simulink model "npc_controller"  (R2022a)
settings: Solver=FixedStepDiscrete  StartTime=0.0  StopTime=20  RelTol=1e-3  EnableMultiTasking=on
undefined symbols (not defined in the file): CAN_O_INT, CANA_BASE, Down, GPTRIP1SEL, GPTRIP2SEL, GPTRIP3SEL, Tsw, TZ1, TZ2, TZ3, Up
libraries: simulink x147, hdlsllib x90, c2802xlib x34, c2837xDlib x20, c280xlib x12, canmsglib x9, c2838xlib x8, idelinklib_common x3, c2806xlib x2, slpidlib x2, c28004xlib x2, c281xlib x2
(part 12 of 42)

== system npc_controller/CONTROL/STATE-MACHINE/CPU_CONTROL_200_A2_precharge_pfc_ok2/updateSequencePhA/pol_ix1 ==
  note: 75dig -> 3iac
  ix : Inport
  Trigger : TriggerPort  TriggerType=function-call  VariantControl=(inherit)  PortDimensions=1
  If : If  IfExpression="(u1 > -8)  & (u1 < 8)"  ElseIfExpressions=u1 >= 8
  Merge : Merge  Inputs=3
  neg : Subsystem  TreatAsAtomicUnit=on
  pos : Subsystem  TreatAsAtomicUnit=on
  zero : Subsystem  TreatAsAtomicUnit=on
  pol_ix : Outport
  wires:
  ix/1 -> If/1
  If/1 -> zero/Action
  zero/1(Out1) -> Merge/1
  If/2 -> pos/Action
  If/3 -> neg/Action
  neg/1(Out1) -> Merge/3
  pos/1(Out1) -> Merge/2
  Merge/1 -> pol_ix/1

== system npc_controller/CONTROL/STATE-MACHINE/CPU_CONTROL_200_A2_precharge_pfc_ok2/updateSequencePhA/pol_vxn1 ==
  note: 16dig -> 5vac
  vxn : Inport
  Trigger : TriggerPort  TriggerType=function-call  VariantControl=(inherit)  PortDimensions=1
  If : If  IfExpression="(u1 > -16)  & (u1 < 16)"  ElseIfExpressions=u1 >= 16
  Merge : Merge  Inputs=3
  neg : Subsystem  TreatAsAtomicUnit=on
  pos : Subsystem  TreatAsAtomicUnit=on
  zero : Subsystem  TreatAsAtomicUnit=on
  pol_vxn : Outport
  wires:
  Merge/1 -> pol_vxn/1
  pos/1(Out1) -> Merge/2
  neg/1(Out1) -> Merge/3
  If/3 -> neg/Action
  If/2 -> pos/Action
  zero/1(Out1) -> Merge/1
  If/1 -> zero/Action
  vxn/1 -> If/1

== system npc_controller/CONTROL/STATE-MACHINE/CPU_CONTROL_200_A2_precharge_pfc_ok2/updateSequencePhB/pol_final1 ==
  vxn : Inport
  ix : Inport  Port=2
  Trigger : TriggerPort  TriggerType=function-call  VariantControl=(inherit)  PortDimensions=1
  If : If  NumInputs=2  IfExpression="((u1 == 1)  & (u2 == 2)) | ((u1 == 2)  & (u2 == 1))"
  Merge : Merge
  pol_vxn : Subsystem  TreatAsAtomicUnit=on
  prot : Subsystem  TreatAsAtomicUnit=on
  pol : Outport
  wires:
  ix/1 -> If/2
  vxn/1 -> pol_vxn/1(vxn), If/1
  Merge/1 -> pol/1
  If/2 -> pol_vxn/Action
  prot/1(Out1) -> Merge/1
  If/1 -> prot/Action
  pol_vxn/1(Out1) -> Merge/2

== system npc_controller/CONTROL/STATE-MACHINE/CPU_CONTROL_200_A2_precharge_pfc_ok2/updateSequencePhB/pol_ix1 ==
  note: 75dig -> 3iac
  ix : Inport
  Trigger : TriggerPort  TriggerType=function-call  VariantControl=(inherit)  PortDimensions=1
  If : If  IfExpression="(u1 > -8)  & (u1 < 8)"  ElseIfExpressions=u1 >= 8
  Merge : Merge  Inputs=3
  neg : Subsystem  TreatAsAtomicUnit=on
  pos : Subsystem  TreatAsAtomicUnit=on
  zero : Subsystem  TreatAsAtomicUnit=on
  pol_ix : Outport
  wires:
  ix/1 -> If/1
  If/1 -> zero/Action
  zero/1(Out1) -> Merge/1
  If/2 -> pos/Action
  If/3 -> neg/Action
  neg/1(Out1) -> Merge/3
  pos/1(Out1) -> Merge/2
  Merge/1 -> pol_ix/1

== system npc_controller/CONTROL/STATE-MACHINE/CPU_CONTROL_200_A2_precharge_pfc_ok2/updateSequencePhB/pol_vxn1 ==
  note: 16dig -> 5vac
  vxn : Inport
  Trigger : TriggerPort  TriggerType=function-call  VariantControl=(inherit)  PortDimensions=1
  If : If  IfExpression="(u1 > -16)  & (u1 < 16)"  ElseIfExpressions=u1 >= 16
  Merge : Merge  Inputs=3
  neg : Subsystem  TreatAsAtomicUnit=on
  pos : Subsystem  TreatAsAtomicUnit=on
  zero : Subsystem  TreatAsAtomicUnit=on
  pol_vxn : Outport
  wires:
  Merge/1 -> pol_vxn/1
  pos/1(Out1) -> Merge/2
  neg/1(Out1) -> Merge/3
  If/3 -> neg/Action
  If/2 -> pos/Action
  zero/1(Out1) -> Merge/1
  If/1 -> zero/Action
  vxn/1 -> If/1

== system npc_controller/CONTROL/STATE-MACHINE/CPU_CONTROL_200_A2_precharge_pfc_ok2/updateSequencePhC/pol_final1 ==
  vxn : Inport
  ix : Inport  Port=2
  Trigger : TriggerPort  TriggerType=function-call  VariantControl=(inherit)  PortDimensions=1
  If : If  NumInputs=2  IfExpression="((u1 == 1)  & (u2 == 2)) | ((u1 == 2)  & (u2 == 1))"
  Merge : Merge
  pol_vxn : Subsystem  TreatAsAtomicUnit=on
  prot : Subsystem  TreatAsAtomicUnit=on
  pol : Outport
  wires:
  ix/1 -> If/2
  vxn/1 -> pol_vxn/1(vxn), If/1
  Merge/1 -> pol/1
  If/2 -> pol_vxn/Action
  prot/1(Out1) -> Merge/1
  If/1 -> prot/Action
  pol_vxn/1(Out1) -> Merge/2

== system npc_controller/CONTROL/STATE-MACHINE/CPU_CONTROL_200_A2_precharge_pfc_ok2/updateSequencePhC/pol_ix1 ==
  note: 75dig -> 3iac
  ix : Inport
  Trigger : TriggerPort  TriggerType=function-call  VariantControl=(inherit)  PortDimensions=1
  If : If  IfExpression="(u1 > -8)  & (u1 < 8)"  ElseIfExpressions=u1 >= 8
  Merge : Merge  Inputs=3
  neg : Subsystem  TreatAsAtomicUnit=on
  pos : Subsystem  TreatAsAtomicUnit=on
  zero : Subsystem  TreatAsAtomicUnit=on
  pol_ix : Outport
  wires:
  ix/1 -> If/1
  If/1 -> zero/Action
  zero/1(Out1) -> Merge/1
  If/2 -> pos/Action
  If/3 -> neg/Action
  neg/1(Out1) -> Merge/3
  pos/1(Out1) -> Merge/2
  Merge/1 -> pol_ix/1

== system npc_controller/CONTROL/STATE-MACHINE/CPU_CONTROL_200_A2_precharge_pfc_ok2/updateSequencePhC/pol_vxn1 ==
  note: 16dig -> 5vac
  vxn : Inport
  Trigger : TriggerPort  TriggerType=function-call  VariantControl=(inherit)  PortDimensions=1
  If : If  IfExpression="(u1 > -16)  & (u1 < 16)"  ElseIfExpressions=u1 >= 16
  Merge : Merge  Inputs=3
  neg : Subsystem  TreatAsAtomicUnit=on
  pos : Subsystem  TreatAsAtomicUnit=on
  zero : Subsystem  TreatAsAtomicUnit=on
  pol_vxn : Outport
  wires:
  Merge/1 -> pol_vxn/1
  pos/1(Out1) -> Merge/2
  neg/1(Out1) -> Merge/3
  If/3 -> neg/Action
  If/2 -> pos/Action
  zero/1(Out1) -> Merge/1
  If/1 -> zero/Action
  vxn/1 -> If/1

== system npc_controller/CONTROL/STATE-MACHINE/CPU_CONTROL_200_A2_precharge_pfc_ok2_OL SS/configFutDis/System Outputs1 ==

== system npc_controller/CONTROL/STATE-MACHINE/CPU_CONTROL_200_A2_precharge_pfc_ok2_OL SS/configFutDis/System Outputs2 ==

== system npc_controller/CONTROL/STATE-MACHINE/CPU_CONTROL_200_A2_precharge_pfc_ok2_OL SS/configFutEn/System Outputs1 ==

== system npc_controller/CONTROL/STATE-MACHINE/CPU_CONTROL_200_A2_precharge_pfc_ok2_OL SS/configFutEn/System Outputs2 ==

== system npc_controller/CONTROL/STATE-MACHINE/CPU_CONTROL_200_A2_precharge_pfc_ok2_OL SS/configFutEn/System Outputs3 ==

== system npc_controller/CONTROL/STATE-MACHINE/CPU_CONTROL_200_A2_precharge_pfc_ok2_OL SS/configGrid/FORCE_TZ ==
  note: 0 - Three phase
      | 1 - Single phase
  In1 : Inport
  sinlgeph_config : Inport  Port=2
  Trigger : TriggerPort  TriggerType=function-call  VariantControl=(inherit)  PortDimensions=1
  1P : Subsystem  TreatAsAtomicUnit=on
  3P3W : Subsystem  TreatAsAtomicUnit=on
  If : If  IfExpression=u1 == 0
  wires:
  If/1 -> 3P3W/Action
  sinlgeph_config/1 -> 1P/1(sinlgeph_config)
  If/2 -> 1P/Action
  In1/1 -> If/1

== system npc_controller/CONTROL/STATE-MACHINE/CPU_CONTROL_200_A2_precharge_pfc_ok2_OL SS/configGrid/RESET_TZ ==
  note: EALLOW;
      |
      | /*Disabled tripzone action*/
      | EPwm6Regs.TZCTL.bit.TZA = (uint16_T)(0b11); //do nothing
      | EPwm6Regs.TZCTL.bit.TZB = (uint16_T)(0b11);
      | EPwm7Regs.TZCTL.bit.TZA = (uint16_T)(0b11);
      | EPwm7Regs.TZCTL.bit.TZB = (uint16_T)(0b11);
      | EPwm8Regs.TZCTL.bit.TZA = (uint16_T)(0b11);
      | EPwm8Regs.TZCTL.bit.TZB = (uint16_T)(0b11);
      | EPwm9Regs.TZCTL.bit.TZA = (uint16_T)(0b11);
      | EPwm9Regs.TZCTL.bit.TZB = (uint16_T)(0b11);
      | EPwm10Regs.TZCTL.bit.TZA = (uint16_T)(0b11);
      | EPwm10Regs.TZCTL.bit.TZB = (uint16_T)(0b11);
      | EPwm11Regs.TZCTL.bit.TZA = (uint16_T)(0b11);
      | EPwm11Regs.TZCTL.bit.TZB = (uint16_T)(0b11);
      |
      | /*Clear grouped OST TZ flags*/
      | EPwm6Regs.TZCLR.bit.OST = 0b1; //clear trip
      | EPwm7Regs.TZCLR.bit.OST = 0b1;
      | EPwm8Regs.TZCLR.bit.OST = 0b1;
      | EPwm9Regs.TZCLR.bit.OST = 0b1;
      | EPwm10Regs.TZCLR.bit.OST = 0b1;
      | EPwm11Regs.TZCLR.bit.OST = 0b1;
      |
      | /*Clear individual OST TZ flags*/
      | EPwm6Regs.TZOSTCLR.bit.OST1 = 0b1; //clear trip
      | EPwm6Regs.TZOSTCLR.bit.OST2 = 0b1;
      | EPwm7Regs.TZOSTCLR.bit.OST1 = 0b1;
      | EPwm7Regs.TZOSTCLR.bit.OST2 = 0b1;
      | EPwm8Regs.TZOSTCLR.bit.OST1 = 0b1;
      | EPwm8Regs.TZOSTCLR.bit.OST2 = 0b1;
      | EPwm9Regs.TZOSTCLR.bit.OST1 = 0b1;
      | EPwm9Regs.TZOSTCLR.bit.OST2 = 0b1;
      | EPwm10Regs.TZOSTCLR.bit.OST1 = 0b1;
      | EPwm10Regs.TZOSTCLR.bit.OST2 = 0b1;
      | EPwm11Regs.TZOSTCLR.bit.OST1 = 0b1;
      | EPwm11Regs.TZOSTCLR.bit.OST2 = 0b1;
      |
      | /*Enable tripzone action*/
      | EPwm6Regs.TZCTL.bit.TZA = (uint16_T)(0b10); //force to LOW
      | EPwm6Regs.TZCTL.bit.TZB = (uint16_T)(0b10);
      | EPwm7Regs.TZCTL.bit.TZA = (uint16_T)(0b10);
      | EPwm7Regs.TZCTL.bit.TZB = (uint16_T)(0b10);
      | EPwm8Regs.TZCTL.bit.TZA = (uint16_T)(0b10);
      | EPwm8Regs.TZCTL.bit.TZB = (uint16_T)(0b10);
      | EPwm9Regs.TZCTL.bit.TZA = (uint16_T)(0b10);
      | EPwm9Regs.TZCTL.bit.TZB = (uint16_T)(0b10);
      | EPwm10Regs.TZCTL.bit.TZA = (uint16_T)(0b10);
      | EPwm10Regs.TZCTL.bit.TZB = (uint16_T)(0b10);
      | EPwm11Regs.TZCTL.bit.TZA = (uint16_T)(0b10);
      | EPwm11Regs.TZCTL.bit.TZB = (uint16_T)(0b10);
      |
      | EDIS;
  note: Note:
      | TZCCTL
      | 0b00 - High impedance
      | 0b01 - Force to HIGH
      | 0b10 - Force to LOW
      | 0b11 - Do nothing
      |
      | AQCSFRC
      | 0b00 - disables forced PWM
      | 0b01 - forces PWM to LOW
      | 0b10 - forces PWM to  HIGH
      |
      | TZFRC.bit.OST
      | 0b0 - Do nothing
      | 0b1 - Force TZ
  Trigger : TriggerPort  TriggerType=function-call  VariantControl=(inherit)  PortDimensions=1
  System Outputs2 : Subsystem  mask(System Outputs){ShowInLibBrowser=0}
      mask prompts: ShowInLibBrowser "Simulink:masks:CustCodeMaskParam1_MP"
      settings: CopyFcn=cccopyfcn(gcb)  OpenFcn=ccopenfcn('System Outputs Function')
      mask Help: eval('feval(''rtwprivate'',''rtwhelpview'',''rtw_sys_outputs_block'')');
      mask Display: disp('System\nOutputs');

== system npc_controller/CONTROL/STATE-MACHINE/CPU_CONTROL_200_A2_precharge_pfc_ok2_OL SS/detectUvpOvp1/False ==
  Action Port : ActionPort
  Constant : Constant  Value=0  OutDataTypeStr=boolean  SampleTime=-1
  low : Outport
  wires:
  Constant/1 -> low/1

== system npc_controller/CONTROL/STATE-MACHINE/CPU_CONTROL_200_A2_precharge_pfc_ok2_OL SS/detectUvpOvp1/True ==
  Action Port : ActionPort
  Constant1 : Constant  OutDataTypeStr=boolean  SampleTime=-1
  high : Outport
  wires:
  Constant1/1 -> high/1

== system npc_controller/CONTROL/STATE-MACHINE/CPU_CONTROL_200_A2_precharge_pfc_ok2_OL SS/detectZCPhA/false ==
  Action Port : ActionPort  ActionPortLabel=else
  Constant1 : Constant  Value=0  OutDataTypeStr=boolean  SampleTime=-1
  ph_en_out : Outport
  wires:
  Constant1/1 -> ph_en_out/1

== system npc_controller/CONTROL/STATE-MACHINE/CPU_CONTROL_200_A2_precharge_pfc_ok2_OL SS/detectZCPhA/true ==
  Action Port : ActionPort  ActionPortLabel="if((u1 > -5)  & (u1 < 5))"
  Constant : Constant  OutDataTypeStr=boolean  SampleTime=-1
  ph_en : Outport
  wires:
  Constant/1 -> ph_en/1

== system npc_controller/CONTROL/STATE-MACHINE/CPU_CONTROL_200_A2_precharge_pfc_ok2_OL SS/detectZCPhB/false ==
  Action Port : ActionPort  ActionPortLabel=else
  Constant1 : Constant  Value=0  OutDataTypeStr=boolean  SampleTime=-1
  ph_en_out : Outport
  wires:
  Constant1/1 -> ph_en_out/1

== system npc_controller/CONTROL/STATE-MACHINE/CPU_CONTROL_200_A2_precharge_pfc_ok2_OL SS/detectZCPhB/true ==
  Action Port : ActionPort  ActionPortLabel="if((u1 > -5)  & (u1 < 5))"
  Constant : Constant  OutDataTypeStr=boolean  SampleTime=-1
  ph_en : Outport
  wires:
  Constant/1 -> ph_en/1

== system npc_controller/CONTROL/STATE-MACHINE/CPU_CONTROL_200_A2_precharge_pfc_ok2_OL SS/detectZCPhC/false ==
  Action Port : ActionPort  ActionPortLabel=else
  Constant1 : Constant  Value=0  OutDataTypeStr=boolean  SampleTime=-1
  ph_en_out : Outport
  wires:
  Constant1/1 -> ph_en_out/1

== system npc_controller/CONTROL/STATE-MACHINE/CPU_CONTROL_200_A2_precharge_pfc_ok2_OL SS/detectZCPhC/true ==
  Action Port : ActionPort  ActionPortLabel="if((u1 > -5)  & (u1 < 5))"
  Constant : Constant  OutDataTypeStr=boolean  SampleTime=-1
  ph_en : Outport
  wires:
  Constant/1 -> ph_en/1

== system npc_controller/CONTROL/STATE-MACHINE/CPU_CONTROL_200_A2_precharge_pfc_ok2_OL SS/disDigCmpMode/System Outputs2 ==

== system npc_controller/CONTROL/STATE-MACHINE/CPU_CONTROL_200_A2_precharge_pfc_ok2_OL SS/disablePwm/System Outputs ==

== system npc_controller/CONTROL/STATE-MACHINE/CPU_CONTROL_200_A2_precharge_pfc_ok2_OL SS/enDigCmpMode/System Outputs2 ==

== system npc_controller/CONTROL/STATE-MACHINE/CPU_CONTROL_200_A2_precharge_pfc_ok2_OL SS/updateCalib/cnt ==
  cnt_calib : Inport  OutDataTypeStr=uint16
  van : Inport  Port=2  OutDataTypeStr=single  PortDimensions=1
  vbn : Inport  Port=3  OutDataTypeStr=single  PortDimensions=1
  vcn : Inport  Port=4  OutDataTypeStr=single  PortDimensions=1
  ia : Inport  Port=5  OutDataTypeStr=single  PortDimensions=1
  ib : Inport  Port=6  OutDataTypeStr=single  PortDimensions=1
  ic : Inport  Port=7  OutDataTypeStr=single  PortDimensions=1
  Action Port : ActionPort  ActionPortLabel=else
  Add : Sum  AccumDataTypeStr=uint16  OutDataTypeStr=uint16
  Constant : Constant  OutDataTypeStr=uint16  SampleTime=-1
  Constant1 : Constant  Value=0  OutDataTypeStr=boolean  SampleTime=-1
  Data Store Write : DataStoreWrite  DataStoreName=adc_offset_ib_tmp  IndexOptions=Index vector (dialog)  Indices=1  OutputSizes=1
  Data Store Write1 : DataStoreWrite  DataStoreName=adc_offset_ic_tmp  IndexOptions=Index vector (dialog)  Indices=1  OutputSizes=1
  Data Store Write2 : DataStoreWrite  DataStoreName=cnt_calib  IndexOptions=Index vector (dialog)  Indices=1  OutputSizes=1
  Data Store Write3 : DataStoreWrite  DataStoreName=adc_offset_vc_tmp  IndexOptions=Index vector (dialog)  Indices=1  OutputSizes=1
  Data Store Write4 : DataStoreWrite  DataStoreName=adc_offset_ia_tmp  IndexOptions=Index vector (dialog)  Indices=1  OutputSizes=1
  Data Store Write5 : DataStoreWrite  DataStoreName=adc_offset_va_tmp  IndexOptions=Index vector (dialog)  Indices=1  OutputSizes=1
  Data Store Write6 : DataStoreWrite  DataStoreName=adc_offset_vb_tmp  IndexOptions=Index vector (dialog)  Indices=1  OutputSizes=1
  IIR Filter2 : Subsystem  Commented=on
  Subsystem1 : Subsystem
  Subsystem2 : Subsystem
  Subsystem3 : Subsystem
  Subsystem4 : Subsystem
  Subsystem5 : Subsystem
  Subsystem6 : Subsystem
  calib_ok : Outport
  wires:
  cnt_calib/1 -> Add/1
  Add/1 -> Data Store Write2/1
  Constant1/1 -> calib_ok/1
  Subsystem2/1(average) -> Data Store Write/1  "va"
  Constant/1 -> Add/2
  Subsystem1/1(average) -> Data Store Write1/1  "va"
  Subsystem3/1(average) -> Data Store Write4/1  "va"
  Subsystem4/1(average) -> Data Store Write3/1  "va"
  Subsystem6/1(average) -> Data Store Write5/1  "va"
  van/1 -> Subsystem6/1(sample)
  Subsystem5/1(average) -> Data Store Write6/1  "va"
  vcn/1 -> Subsystem4/1(sample)
  vbn/1 -> Subsystem5/1(sample)
  ia/1 -> Subsystem3/1(sample)
  ic/1 -> Subsystem1/1(sample)
  ib/1 -> Subsystem2/1(sample)

== system npc_controller/CONTROL/STATE-MACHINE/CPU_CONTROL_200_A2_precharge_pfc_ok2_OL SS/updateCalib/done ==
  Action Port : ActionPort  ActionPortLabel=if(u1 > 65000)
  AUTO-CALIB_DONE : Subsystem
  CLEAR_FAULTS : Subsystem
  Function-Call Generator : simulink/Ports & Subsystems/Function-Call Generator  sample_time=-1  numberOfIterations=1  DisallowWideOutput=off
  Function-Call Split1 : FunctionCallSplit  NumOutputPorts=2
  Function-Call Split2 : FunctionCallSplit  NumOutputPorts=2
  RESET_TZ : Subsystem
  calib_ok : Outport
  wires:
  Function-Call Generator/1 -> Function-Call Split1/1
  Function-Call Split1/2 -> Function-Call Split2/1
  AUTO-CALIB_DONE/1(Out1) -> calib_ok/1
  Function-Call Split1/1 -> AUTO-CALIB_DONE/Trigger
  Function-Call Split2/1 -> RESET_TZ/Trigger
  Function-Call Split2/2 -> CLEAR_FAULTS/Trigger

== system npc_controller/CONTROL/STATE-MACHINE/CPU_CONTROL_200_A2_precharge_pfc_ok2_OL SS/updatePll3p/PLL ==
  abc : Inport
  Demux : Demux  Commented=on  Outputs=3
  If1 : If  Commented=on  IfExpression=(u1 > 0)  ShowElse=off
  SRF_PLL : Subsystem
  Subsystem : Subsystem  Commented=on
  theta : Outport  OutDataTypeStr=single
  wires:
  SRF_PLL/3(theta) -> theta/1
  Subsystem/1(Out1) -> If1/1
  abc/1 -> SRF_PLL/1(Vabc), Demux/1
  Demux/1 -> Subsystem/1(In1)

== system npc_controller/CONTROL/STATE-MACHINE/CPU_CONTROL_200_A2_precharge_pfc_ok2_OL SS/updateSequencePhA/pol_final1 ==
  vxn : Inport
  ix : Inport  Port=2
  Trigger : TriggerPort  TriggerType=function-call  VariantControl=(inherit)  PortDimensions=1
  If : If  NumInputs=2  IfExpression="((u1 == 1)  & (u2 == 2)) | ((u1 == 2)  & (u2 == 1))"
  Merge : Merge
  pol_vxn : Subsystem  TreatAsAtomicUnit=on
  prot : Subsystem  TreatAsAtomicUnit=on
  pol : Outport
  wires:
  ix/1 -> If/2
  vxn/1 -> pol_vxn/1(vxn), If/1
  Merge/1 -> pol/1
  If/2 -> pol_vxn/Action
  prot/1(Out1) -> Merge/1
  If/1 -> prot/Action
  pol_vxn/1(Out1) -> Merge/2

== system npc_controller/CONTROL/STATE-MACHINE/CPU_CONTROL_200_A2_precharge_pfc_ok2_OL SS/updateSequencePhA/pol_ix1 ==
  note: 75dig -> 3iac
  ix : Inport
  Trigger : TriggerPort  TriggerType=function-call  VariantControl=(inherit)  PortDimensions=1
  If : If  IfExpression="(u1 > -8)  & (u1 < 8)"  ElseIfExpressions=u1 >= 8
  Merge : Merge  Inputs=3
  neg : Subsystem  TreatAsAtomicUnit=on
  pos : Subsystem  TreatAsAtomicUnit=on
  zero : Subsystem  TreatAsAtomicUnit=on
  pol_ix : Outport
  wires:
  ix/1 -> If/1
  If/1 -> zero/Action
  zero/1(Out1) -> Merge/1
  If/2 -> pos/Action
  If/3 -> neg/Action
  neg/1(Out1) -> Merge/3
  pos/1(Out1) -> Merge/2
  Merge/1 -> pol_ix/1

== system npc_controller/CONTROL/STATE-MACHINE/CPU_CONTROL_200_A2_precharge_pfc_ok2_OL SS/updateSequencePhA/pol_vxn1 ==
  note: 16dig -> 5vac
  vxn : Inport
  Trigger : TriggerPort  TriggerType=function-call  VariantControl=(inherit)  PortDimensions=1
  If : If  IfExpression="(u1 > -16)  & (u1 < 16)"  ElseIfExpressions=u1 >= 16
  Merge : Merge  Inputs=3
  neg : Subsystem  TreatAsAtomicUnit=on
  pos : Subsystem  TreatAsAtomicUnit=on
  zero : Subsystem  TreatAsAtomicUnit=on
  pol_vxn : Outport
  wires:
  Merge/1 -> pol_vxn/1
  pos/1(Out1) -> Merge/2
  neg/1(Out1) -> Merge/3
  If/3 -> neg/Action
  If/2 -> pos/Action
  zero/1(Out1) -> Merge/1
  If/1 -> zero/Action
  vxn/1 -> If/1

== system npc_controller/CONTROL/STATE-MACHINE/CPU_CONTROL_200_A2_precharge_pfc_ok2_OL SS/updateSequencePhB/pol_final1 ==
  vxn : Inport
  ix : Inport  Port=2
  Trigger : TriggerPort  TriggerType=function-call  VariantControl=(inherit)  PortDimensions=1
  If : If  NumInputs=2  IfExpression="((u1 == 1)  & (u2 == 2)) | ((u1 == 2)  & (u2 == 1))"
  Merge : Merge
  pol_vxn : Subsystem  TreatAsAtomicUnit=on
  prot : Subsystem  TreatAsAtomicUnit=on
  pol : Outport
  wires:
  ix/1 -> If/2
  vxn/1 -> pol_vxn/1(vxn), If/1
  Merge/1 -> pol/1
  If/2 -> pol_vxn/Action
  prot/1(Out1) -> Merge/1
  If/1 -> prot/Action
  pol_vxn/1(Out1) -> Merge/2

== system npc_controller/CONTROL/STATE-MACHINE/CPU_CONTROL_200_A2_precharge_pfc_ok2_OL SS/updateSequencePhB/pol_ix1 ==
  note: 75dig -> 3iac
  ix : Inport
  Trigger : TriggerPort  TriggerType=function-call  VariantControl=(inherit)  PortDimensions=1
  If : If  IfExpression="(u1 > -8)  & (u1 < 8)"  ElseIfExpressions=u1 >= 8
  Merge : Merge  Inputs=3
  neg : Subsystem  TreatAsAtomicUnit=on
  pos : Subsystem  TreatAsAtomicUnit=on
  zero : Subsystem  TreatAsAtomicUnit=on
  pol_ix : Outport
  wires:
  ix/1 -> If/1
  If/1 -> zero/Action
  zero/1(Out1) -> Merge/1
  If/2 -> pos/Action
  If/3 -> neg/Action
  neg/1(Out1) -> Merge/3
  pos/1(Out1) -> Merge/2
  Merge/1 -> pol_ix/1

== system npc_controller/CONTROL/STATE-MACHINE/CPU_CONTROL_200_A2_precharge_pfc_ok2_OL SS/updateSequencePhB/pol_vxn1 ==
  note: 16dig -> 5vac
  vxn : Inport
  Trigger : TriggerPort  TriggerType=function-call  VariantControl=(inherit)  PortDimensions=1
  If : If  IfExpression="(u1 > -16)  & (u1 < 16)"  ElseIfExpressions=u1 >= 16
  Merge : Merge  Inputs=3
  neg : Subsystem  TreatAsAtomicUnit=on
  pos : Subsystem  TreatAsAtomicUnit=on
  zero : Subsystem  TreatAsAtomicUnit=on
  pol_vxn : Outport
  wires:
  Merge/1 -> pol_vxn/1
  pos/1(Out1) -> Merge/2
  neg/1(Out1) -> Merge/3
  If/3 -> neg/Action
  If/2 -> pos/Action
  zero/1(Out1) -> Merge/1
  If/1 -> zero/Action
  vxn/1 -> If/1

== system npc_controller/CONTROL/STATE-MACHINE/CPU_CONTROL_200_A2_precharge_pfc_ok2_OL SS/updateSequencePhC/pol_final1 ==
  vxn : Inport
  ix : Inport  Port=2
  Trigger : TriggerPort  TriggerType=function-call  VariantControl=(inherit)  PortDimensions=1
  If : If  NumInputs=2  IfExpression="((u1 == 1)  & (u2 == 2)) | ((u1 == 2)  & (u2 == 1))"
  Merge : Merge
  pol_vxn : Subsystem  TreatAsAtomicUnit=on
  prot : Subsystem  TreatAsAtomicUnit=on
  pol : Outport
  wires:
  ix/1 -> If/2
  vxn/1 -> pol_vxn/1(vxn), If/1
  Merge/1 -> pol/1
  If/2 -> pol_vxn/Action
  prot/1(Out1) -> Merge/1
  If/1 -> prot/Action
  pol_vxn/1(Out1) -> Merge/2

== system npc_controller/CONTROL/STATE-MACHINE/CPU_CONTROL_200_A2_precharge_pfc_ok2_OL SS/updateSequencePhC/pol_ix1 ==
  note: 75dig -> 3iac
  ix : Inport
  Trigger : TriggerPort  TriggerType=function-call  VariantControl=(inherit)  PortDimensions=1
  If : If  IfExpression="(u1 > -8)  & (u1 < 8)"  ElseIfExpressions=u1 >= 8
  Merge : Merge  Inputs=3
  neg : Subsystem  TreatAsAtomicUnit=on
  pos : Subsystem  TreatAsAtomicUnit=on
  zero : Subsystem  TreatAsAtomicUnit=on
  pol_ix : Outport
  wires:
  ix/1 -> If/1
  If/1 -> zero/Action
  zero/1(Out1) -> Merge/1
  If/2 -> pos/Action
  If/3 -> neg/Action
  neg/1(Out1) -> Merge/3
  pos/1(Out1) -> Merge/2
  Merge/1 -> pol_ix/1

== system npc_controller/CONTROL/STATE-MACHINE/CPU_CONTROL_200_A2_precharge_pfc_ok2_OL SS/updateSequencePhC/pol_vxn1 ==
  note: 16dig -> 5vac
  vxn : Inport
  Trigger : TriggerPort  TriggerType=function-call  VariantControl=(inherit)  PortDimensions=1
  If : If  IfExpression="(u1 > -16)  & (u1 < 16)"  ElseIfExpressions=u1 >= 16
  Merge : Merge  Inputs=3
  neg : Subsystem  TreatAsAtomicUnit=on
  pos : Subsystem  TreatAsAtomicUnit=on
  zero : Subsystem  TreatAsAtomicUnit=on
  pol_vxn : Outport
  wires:
  Merge/1 -> pol_vxn/1
  pos/1(Out1) -> Merge/2
  neg/1(Out1) -> Merge/3
  If/3 -> neg/Action
  If/2 -> pos/Action
  zero/1(Out1) -> Merge/1
  If/1 -> zero/Action
  vxn/1 -> If/1

== system npc_controller/CONTROL/STATE-MACHINE/CPU_CONTROL_200_A2_precharge_pfc_ok2_OL SS1/ClrCmpssTz/System Outputs1 ==

== system npc_controller/CONTROL/STATE-MACHINE/CPU_CONTROL_200_A2_precharge_pfc_ok2_OL SS1/ClrCmpssTz/System Outputs2 ==

== system npc_controller/CONTROL/STATE-MACHINE/CPU_CONTROL_200_A2_precharge_pfc_ok2_OL SS1/configFutDis/System Outputs1 ==

== system npc_controller/CONTROL/STATE-MACHINE/CPU_CONTROL_200_A2_precharge_pfc_ok2_OL SS1/configFutDis/System Outputs2 ==

== system npc_controller/CONTROL/STATE-MACHINE/CPU_CONTROL_200_A2_precharge_pfc_ok2_OL SS1/configFutEn/System Outputs1 ==

== system npc_controller/CONTROL/STATE-MACHINE/CPU_CONTROL_200_A2_precharge_pfc_ok2_OL SS1/configFutEn/System Outputs2 ==

== system npc_controller/CONTROL/STATE-MACHINE/CPU_CONTROL_200_A2_precharge_pfc_ok2_OL SS1/configFutEn/System Outputs3 ==

== system npc_controller/CONTROL/STATE-MACHINE/CPU_CONTROL_200_A2_precharge_pfc_ok2_OL SS1/configGrid/FORCE_TZ ==
  note: 0 - Three phase
      | 1 - Single phase
  In1 : Inport
  sinlgeph_config : Inport  Port=2
  Trigger : TriggerPort  TriggerType=function-call  VariantControl=(inherit)  PortDimensions=1
  1P : Subsystem  TreatAsAtomicUnit=on
  3P3W : Subsystem  TreatAsAtomicUnit=on
  If : If  IfExpression=u1 == 0
  wires:
  In1/1 -> If/1
  If/2 -> 1P/Action
  sinlgeph_config/1 -> 1P/1(sinlgeph_config)
  If/1 -> 3P3W/Action

== system npc_controller/CONTROL/STATE-MACHINE/CPU_CONTROL_200_A2_precharge_pfc_ok2_OL SS1/configGrid/RESET_TZ ==
  note: Note:
      | TZCCTL
      | 0b00 - High impedance
      | 0b01 - Force to HIGH
      | 0b10 - Force to LOW
      | 0b11 - Do nothing
      |
      | AQCSFRC
      | 0b00 - disables forced PWM
      | 0b01 - forces PWM to LOW
      | 0b10 - forces PWM to  HIGH
      |
      | TZFRC.bit.OST
      | 0b0 - Do nothing
      | 0b1 - Force TZ
  note: EALLOW;
      |
      | /*Disabled tripzone action*/
      | EPwm6Regs.TZCTL.bit.TZA = (uint16_T)(0b11); //do nothing
      | EPwm6Regs.TZCTL.bit.TZB = (uint16_T)(0b11);
      | EPwm7Regs.TZCTL.bit.TZA = (uint16_T)(0b11);
      | EPwm7Regs.TZCTL.bit.TZB = (uint16_T)(0b11);
      | EPwm8Regs.TZCTL.bit.TZA = (uint16_T)(0b11);
      | EPwm8Regs.TZCTL.bit.TZB = (uint16_T)(0b11);
      | EPwm9Regs.TZCTL.bit.TZA = (uint16_T)(0b11);
      | EPwm9Regs.TZCTL.bit.TZB = (uint16_T)(0b11);
      | EPwm10Regs.TZCTL.bit.TZA = (uint16_T)(0b11);
      | EPwm10Regs.TZCTL.bit.TZB = (uint16_T)(0b11);
      | EPwm11Regs.TZCTL.bit.TZA = (uint16_T)(0b11);
      | EPwm11Regs.TZCTL.bit.TZB = (uint16_T)(0b11);
      |
      | /*Clear grouped OST TZ flags*/
      | EPwm6Regs.TZCLR.bit.OST = 0b1; //clear trip
      | EPwm7Regs.TZCLR.bit.OST = 0b1;
      | EPwm8Regs.TZCLR.bit.OST = 0b1;
      | EPwm9Regs.TZCLR.bit.OST = 0b1;
      | EPwm10Regs.TZCLR.bit.OST = 0b1;
      | EPwm11Regs.TZCLR.bit.OST = 0b1;
      |
      | /*Clear individual OST TZ flags*/
      | EPwm6Regs.TZOSTCLR.bit.OST1 = 0b1; //clear trip
      | EPwm6Regs.TZOSTCLR.bit.OST2 = 0b1;
      | EPwm7Regs.TZOSTCLR.bit.OST1 = 0b1;
      | EPwm7Regs.TZOSTCLR.bit.OST2 = 0b1;
      | EPwm8Regs.TZOSTCLR.bit.OST1 = 0b1;
      | EPwm8Regs.TZOSTCLR.bit.OST2 = 0b1;
      | EPwm9Regs.TZOSTCLR.bit.OST1 = 0b1;
      | EPwm9Regs.TZOSTCLR.bit.OST2 = 0b1;
      | EPwm10Regs.TZOSTCLR.bit.OST1 = 0b1;
      | EPwm10Regs.TZOSTCLR.bit.OST2 = 0b1;
      | EPwm11Regs.TZOSTCLR.bit.OST1 = 0b1;
      | EPwm11Regs.TZOSTCLR.bit.OST2 = 0b1;
      |
      | /*Enable tripzone action*/
      | EPwm6Regs.TZCTL.bit.TZA = (uint16_T)(0b10); //force to LOW
      | EPwm6Regs.TZCTL.bit.TZB = (uint16_T)(0b10);
      | EPwm7Regs.TZCTL.bit.TZA = (uint16_T)(0b10);
      | EPwm7Regs.TZCTL.bit.TZB = (uint16_T)(0b10);
      | EPwm8Regs.TZCTL.bit.TZA = (uint16_T)(0b10);
      | EPwm8Regs.TZCTL.bit.TZB = (uint16_T)(0b10);
      | EPwm9Regs.TZCTL.bit.TZA = (uint16_T)(0b10);
      | EPwm9Regs.TZCTL.bit.TZB = (uint16_T)(0b10);
      | EPwm10Regs.TZCTL.bit.TZA = (uint16_T)(0b10);
      | EPwm10Regs.TZCTL.bit.TZB = (uint16_T)(0b10);
      | EPwm11Regs.TZCTL.bit.TZA = (uint16_T)(0b10);
      | EPwm11Regs.TZCTL.bit.TZB = (uint16_T)(0b10);
      |
      | EDIS;
  Trigger : TriggerPort  TriggerType=function-call  VariantControl=(inherit)  PortDimensions=1
  System Outputs2 : Subsystem  mask(System Outputs){ShowInLibBrowser=0}
      mask prompts: ShowInLibBrowser "Simulink:masks:CustCodeMaskParam1_MP"
      settings: CopyFcn=cccopyfcn(gcb)  OpenFcn=ccopenfcn('System Outputs Function')
      mask Help: eval('feval(''rtwprivate'',''rtwhelpview'',''rtw_sys_outputs_block'')');
      mask Display: disp('System\nOutputs');

== system npc_controller/CONTROL/STATE-MACHINE/CPU_CONTROL_200_A2_precharge_pfc_ok2_OL SS1/detectZCPhA/false ==
  Action Port : ActionPort  ActionPortLabel=else
  Constant1 : Constant  Value=0  OutDataTypeStr=boolean  SampleTime=-1
  ph_en_out : Outport
  wires:
  Constant1/1 -> ph_en_out/1

== system npc_controller/CONTROL/STATE-MACHINE/CPU_CONTROL_200_A2_precharge_pfc_ok2_OL SS1/detectZCPhA/true ==
  Action Port : ActionPort  ActionPortLabel="if((u1 > -5)  & (u1 < 5))"
  Constant : Constant  OutDataTypeStr=boolean  SampleTime=-1
  ph_en : Outport
  wires:
  Constant/1 -> ph_en/1

== system npc_controller/CONTROL/STATE-MACHINE/CPU_CONTROL_200_A2_precharge_pfc_ok2_OL SS1/detectZCPhB/false ==
  Action Port : ActionPort  ActionPortLabel=else
  Constant1 : Constant  Value=0  OutDataTypeStr=boolean  SampleTime=-1
  ph_en_out : Outport
  wires:
  Constant1/1 -> ph_en_out/1

== system npc_controller/CONTROL/STATE-MACHINE/CPU_CONTROL_200_A2_precharge_pfc_ok2_OL SS1/detectZCPhB/true ==
  Action Port : ActionPort  ActionPortLabel="if((u1 > -5)  & (u1 < 5))"
  Constant : Constant  OutDataTypeStr=boolean  SampleTime=-1
  ph_en : Outport
  wires:
  Constant/1 -> ph_en/1

== system npc_controller/CONTROL/STATE-MACHINE/CPU_CONTROL_200_A2_precharge_pfc_ok2_OL SS1/detectZCPhC/false ==
  Action Port : ActionPort  ActionPortLabel=else
  Constant1 : Constant  Value=0  OutDataTypeStr=boolean  SampleTime=-1
  ph_en_out : Outport
  wires:
  Constant1/1 -> ph_en_out/1

== system npc_controller/CONTROL/STATE-MACHINE/CPU_CONTROL_200_A2_precharge_pfc_ok2_OL SS1/detectZCPhC/true ==
  Action Port : ActionPort  ActionPortLabel="if((u1 > -5)  & (u1 < 5))"
  Constant : Constant  OutDataTypeStr=boolean  SampleTime=-1
  ph_en : Outport
  wires:
  Constant/1 -> ph_en/1

== system npc_controller/CONTROL/STATE-MACHINE/CPU_CONTROL_200_A2_precharge_pfc_ok2_OL SS1/disCmpssTz/System Outputs1 ==

== system npc_controller/CONTROL/STATE-MACHINE/CPU_CONTROL_200_A2_precharge_pfc_ok2_OL SS1/disCmpssTz/System Outputs2 ==

== system npc_controller/CONTROL/STATE-MACHINE/CPU_CONTROL_200_A2_precharge_pfc_ok2_OL SS1/disablePwm/System Outputs ==

== system npc_controller/CONTROL/STATE-MACHINE/CPU_CONTROL_200_A2_precharge_pfc_ok2_OL SS1/readCmpssOcp/System Outputs1 ==

== system npc_controller/CONTROL/STATE-MACHINE/CPU_CONTROL_200_A2_precharge_pfc_ok2_OL SS1/updateCalib/cnt ==
  cnt_calib : Inport  OutDataTypeStr=uint16
  van : Inport  Port=2  OutDataTypeStr=single  PortDimensions=1
  vbn : Inport  Port=3  OutDataTypeStr=single  PortDimensions=1
  vcn : Inport  Port=4  OutDataTypeStr=single  PortDimensions=1
  ia : Inport  Port=5  OutDataTypeStr=single  PortDimensions=1
  ib : Inport  Port=6  OutDataTypeStr=single  PortDimensions=1
  ic : Inport  Port=7  OutDataTypeStr=single  PortDimensions=1
  Action Port : ActionPort  ActionPortLabel=else
  Add : Sum  AccumDataTypeStr=uint16  OutDataTypeStr=uint16
  Constant : Constant  OutDataTypeStr=uint16  SampleTime=-1
  Constant1 : Constant  Value=0  OutDataTypeStr=boolean  SampleTime=-1
  Data Store Write : DataStoreWrite  DataStoreName=adc_offset_ib_tmp  IndexOptions=Index vector (dialog)  Indices=1  OutputSizes=1
  Data Store Write1 : DataStoreWrite  DataStoreName=adc_offset_ic_tmp  IndexOptions=Index vector (dialog)  Indices=1  OutputSizes=1
  Data Store Write2 : DataStoreWrite  DataStoreName=cnt_calib  IndexOptions=Index vector (dialog)  Indices=1  OutputSizes=1
  Data Store Write3 : DataStoreWrite  DataStoreName=adc_offset_vc_tmp  IndexOptions=Index vector (dialog)  Indices=1  OutputSizes=1
  Data Store Write4 : DataStoreWrite  DataStoreName=adc_offset_ia_tmp  IndexOptions=Index vector (dialog)  Indices=1  OutputSizes=1
  Data Store Write5 : DataStoreWrite  DataStoreName=adc_offset_va_tmp  IndexOptions=Index vector (dialog)  Indices=1  OutputSizes=1
  Data Store Write6 : DataStoreWrite  DataStoreName=adc_offset_vb_tmp  IndexOptions=Index vector (dialog)  Indices=1  OutputSizes=1
  IIR Filter2 : Subsystem  Commented=on
  Subsystem1 : Subsystem
  Subsystem2 : Subsystem
  Subsystem3 : Subsystem
  Subsystem4 : Subsystem
  Subsystem5 : Subsystem
  Subsystem6 : Subsystem
  calib_ok : Outport
  wires:
  ib/1 -> Subsystem2/1(sample)
  ic/1 -> Subsystem1/1(sample)
  ia/1 -> Subsystem3/1(sample)
  vbn/1 -> Subsystem5/1(sample)
  vcn/1 -> Subsystem4/1(sample)
  Subsystem5/1(average) -> Data Store Write6/1  "va"
  van/1 -> Subsystem6/1(sample)
  Subsystem6/1(average) -> Data Store Write5/1  "va"
  Subsystem4/1(average) -> Data Store Write3/1  "va"
  Subsystem3/1(average) -> Data Store Write4/1  "va"
  Subsystem1/1(average) -> Data Store Write1/1  "va"
  Constant/1 -> Add/2
  Subsystem2/1(average) -> Data Store Write/1  "va"
  Constant1/1 -> calib_ok/1
  Add/1 -> Data Store Write2/1
  cnt_calib/1 -> Add/1

== system npc_controller/CONTROL/STATE-MACHINE/CPU_CONTROL_200_A2_precharge_pfc_ok2_OL SS1/updateCalib/done ==
  Action Port : ActionPort  ActionPortLabel=if(u1 > 65000)
  AUTO-CALIB_DONE : Subsystem
  CLEAR_FAULTS : Subsystem
  Function-Call Generator : simulink/Ports & Subsystems/Function-Call Generator  sample_time=-1  numberOfIterations=1  DisallowWideOutput=off
  Function-Call Split1 : FunctionCallSplit  NumOutputPorts=2
  Function-Call Split2 : FunctionCallSplit  NumOutputPorts=2
  RESET_TZ : Subsystem
  calib_ok : Outport
  wires:
  Function-Call Split2/2 -> CLEAR_FAULTS/Trigger
  Function-Call Split2/1 -> RESET_TZ/Trigger
  Function-Call Split1/1 -> AUTO-CALIB_DONE/Trigger
  AUTO-CALIB_DONE/1(Out1) -> calib_ok/1
  Function-Call Split1/2 -> Function-Call Split2/1
  Function-Call Generator/1 -> Function-Call Split1/1

== system npc_controller/CONTROL/STATE-MACHINE/CPU_CONTROL_200_A2_precharge_pfc_ok2_OL SS1/updatePll3p/PLL ==
  abc : Inport
  Demux : Demux  Commented=on  Outputs=3
  If1 : If  Commented=on  IfExpression=(u1 > 0)  ShowElse=off
  SRF_PLL : Subsystem
  Subsystem : Subsystem  Commented=on
  theta : Outport  OutDataTypeStr=single
  wires:
  Demux/1 -> Subsystem/1(In1)
  abc/1 -> Demux/1, SRF_PLL/1(Vabc)
  Subsystem/1(Out1) -> If1/1
  SRF_PLL/3(theta) -> theta/1

== system npc_controller/CONTROL/STATE-MACHINE/CPU_CONTROL_200_A2_precharge_pfc_ok2_OL SS1/updateSequencePhA/pol_final1 ==
  vxn : Inport
  ix : Inport  Port=2
  Trigger : TriggerPort  TriggerType=function-call  VariantControl=(inherit)  PortDimensions=1
  If : If  NumInputs=2  IfExpression="((u1 == 1)  & (u2 == 2)) | ((u1 == 2)  & (u2 == 1))"
  Merge : Merge
  pol_vxn : Subsystem  TreatAsAtomicUnit=on
  prot : Subsystem  TreatAsAtomicUnit=on
  pol : Outport
  wires:
  pol_vxn/1(Out1) -> Merge/2
  If/1 -> prot/Action
  prot/1(Out1) -> Merge/1
  If/2 -> pol_vxn/Action
  Merge/1 -> pol/1
  vxn/1 -> If/1, pol_vxn/1(vxn)
  ix/1 -> If/2

== system npc_controller/CONTROL/STATE-MACHINE/CPU_CONTROL_200_A2_precharge_pfc_ok2_OL SS1/updateSequencePhA/pol_ix1 ==
  note: 75dig -> 3iac
  ix : Inport
  Trigger : TriggerPort  TriggerType=function-call  VariantControl=(inherit)  PortDimensions=1
  If : If  IfExpression="(u1 > -8)  & (u1 < 8)"  ElseIfExpressions=u1 >= 8
  Merge : Merge  Inputs=3
  neg : Subsystem  TreatAsAtomicUnit=on
  pos : Subsystem  TreatAsAtomicUnit=on
  zero : Subsystem  TreatAsAtomicUnit=on
  pol_ix : Outport
  wires:
  Merge/1 -> pol_ix/1
  pos/1(Out1) -> Merge/2
  neg/1(Out1) -> Merge/3
  If/3 -> neg/Action
  If/2 -> pos/Action
  zero/1(Out1) -> Merge/1
  If/1 -> zero/Action
  ix/1 -> If/1

== system npc_controller/CONTROL/STATE-MACHINE/CPU_CONTROL_200_A2_precharge_pfc_ok2_OL SS1/updateSequencePhA/pol_vxn1 ==
  note: 16dig -> 5vac
  vxn : Inport
  ixn1 : Inport  Port=2
  Trigger : TriggerPort  TriggerType=function-call  VariantControl=(inherit)  PortDimensions=1
  If : If  IfExpression="(u1 > -16)  & (u1 < 16)"  ElseIfExpressions=u1 >= 16
  Merge : Merge  Inputs=3
  neg : Subsystem  TreatAsAtomicUnit=on
  pos : Subsystem  TreatAsAtomicUnit=on
  zero : Subsystem  TreatAsAtomicUnit=on
  pol_vxn : Outport
  wires:
  vxn/1 -> If/1
  If/1 -> zero/Action
  zero/1(Out1) -> Merge/1
  If/2 -> pos/Action
  If/3 -> neg/Action
  neg/1(Out1) -> Merge/3
  pos/1(Out1) -> Merge/2
  Merge/1 -> pol_vxn/1
  ixn1/1 -> neg/1(ixn), pos/1(ixn)

== system npc_controller/CONTROL/STATE-MACHINE/CPU_CONTROL_200_A2_precharge_pfc_ok2_OL SS1/updateSequencePhA/pol_vxn2 ==
  note: 16dig -> 5vac
  vxn : Inport
  Trigger : TriggerPort  TriggerType=function-call  VariantControl=(inherit)  PortDimensions=1
  If : If  IfExpression="(u1 > -16)  & (u1 < 16)"  ElseIfExpressions=u1 >= 16
  Merge : Merge  Inputs=3
  neg : Subsystem  TreatAsAtomicUnit=on
  pos : Subsystem  TreatAsAtomicUnit=on
  zero : Subsystem  TreatAsAtomicUnit=on
  pol_vxn : Outport
  wires:
  Merge/1 -> pol_vxn/1
  pos/1(Out1) -> Merge/2
  neg/1(Out1) -> Merge/3
  If/3 -> neg/Action
  If/2 -> pos/Action
  zero/1(Out1) -> Merge/1
  If/1 -> zero/Action
  vxn/1 -> If/1

== system npc_controller/CONTROL/STATE-MACHINE/CPU_CONTROL_200_A2_precharge_pfc_ok2_OL SS1/updateSequencePhB/pol_final1 ==
  vxn : Inport
  ix : Inport  Port=2
  Trigger : TriggerPort  TriggerType=function-call  VariantControl=(inherit)  PortDimensions=1
  If : If  NumInputs=2  IfExpression="((u1 == 1)  & (u2 == 2)) | ((u1 == 2)  & (u2 == 1))"
  Merge : Merge
  pol_vxn : Subsystem  TreatAsAtomicUnit=on
  prot : Subsystem  TreatAsAtomicUnit=on
  pol : Outport
  wires:
  pol_vxn/1(Out1) -> Merge/2
  If/1 -> prot/Action
  prot/1(Out1) -> Merge/1
  If/2 -> pol_vxn/Action
  Merge/1 -> pol/1
  vxn/1 -> If/1, pol_vxn/1(vxn)
  ix/1 -> If/2

== system npc_controller/CONTROL/STATE-MACHINE/CPU_CONTROL_200_A2_precharge_pfc_ok2_OL SS1/updateSequencePhB/pol_ix1 ==
  note: 75dig -> 3iac
  ix : Inport
  Trigger : TriggerPort  TriggerType=function-call  VariantControl=(inherit)  PortDimensions=1
  If : If  IfExpression="(u1 > -8)  & (u1 < 8)"  ElseIfExpressions=u1 >= 8
  Merge : Merge  Inputs=3
  neg : Subsystem  TreatAsAtomicUnit=on
  pos : Subsystem  TreatAsAtomicUnit=on
  zero : Subsystem  TreatAsAtomicUnit=on
  pol_ix : Outport
  wires:
  Merge/1 -> pol_ix/1
  pos/1(Out1) -> Merge/2
  neg/1(Out1) -> Merge/3
  If/3 -> neg/Action
  If/2 -> pos/Action
  zero/1(Out1) -> Merge/1
  If/1 -> zero/Action
  ix/1 -> If/1

== system npc_controller/CONTROL/STATE-MACHINE/CPU_CONTROL_200_A2_precharge_pfc_ok2_OL SS1/updateSequencePhB/pol_vxn1 ==
  note: 16dig -> 5vac
  vxn : Inport
  ixn1 : Inport  Port=2
  Trigger : TriggerPort  TriggerType=function-call  VariantControl=(inherit)  PortDimensions=1
  If : If  IfExpression="(u1 > -16)  & (u1 < 16)"  ElseIfExpressions=u1 >= 16
  Merge : Merge  Inputs=3
  neg : Subsystem  TreatAsAtomicUnit=on
  pos : Subsystem  TreatAsAtomicUnit=on
  zero : Subsystem  TreatAsAtomicUnit=on
  pol_vxn : Outport
  wires:
  vxn/1 -> If/1
  If/1 -> zero/Action
  zero/1(Out1) -> Merge/1
  If/2 -> pos/Action
  neg/1(Out1) -> Merge/3
  pos/1(Out1) -> Merge/2
  Merge/1 -> pol_vxn/1
  ixn1/1 -> neg/1(ixn), pos/1(ixn)
  If/3 -> neg/Action

== system npc_controller/CONTROL/STATE-MACHINE/CPU_CONTROL_200_A2_precharge_pfc_ok2_OL SS1/updateSequencePhB/pol_vxn2 ==
  note: 16dig -> 5vac
  vxn : Inport
  Trigger : TriggerPort  TriggerType=function-call  VariantControl=(inherit)  PortDimensions=1
  If : If  IfExpression="(u1 > -16)  & (u1 < 16)"  ElseIfExpressions=u1 >= 16
  Merge : Merge  Inputs=3
  neg : Subsystem  TreatAsAtomicUnit=on
  pos : Subsystem  TreatAsAtomicUnit=on
  zero : Subsystem  TreatAsAtomicUnit=on
  pol_vxn : Outport
  wires:
  Merge/1 -> pol_vxn/1
  pos/1(Out1) -> Merge/2
  neg/1(Out1) -> Merge/3
  If/3 -> neg/Action
  If/2 -> pos/Action
  zero/1(Out1) -> Merge/1
  If/1 -> zero/Action
  vxn/1 -> If/1

== system npc_controller/CONTROL/STATE-MACHINE/CPU_CONTROL_200_A2_precharge_pfc_ok2_OL SS1/updateSequencePhC/pol_final1 ==
  vxn : Inport
  ix : Inport  Port=2
  Trigger : TriggerPort  TriggerType=function-call  VariantControl=(inherit)  PortDimensions=1
  If : If  NumInputs=2  IfExpression="((u1 == 1)  & (u2 == 2)) | ((u1 == 2)  & (u2 == 1))"
  Merge : Merge
  pol_vxn : Subsystem  TreatAsAtomicUnit=on
  prot : Subsystem  TreatAsAtomicUnit=on
  pol : Outport
  wires:
  pol_vxn/1(Out1) -> Merge/2
  If/1 -> prot/Action
  prot/1(Out1) -> Merge/1
  If/2 -> pol_vxn/Action
  Merge/1 -> pol/1
  vxn/1 -> If/1, pol_vxn/1(vxn)
  ix/1 -> If/2

== system npc_controller/CONTROL/STATE-MACHINE/CPU_CONTROL_200_A2_precharge_pfc_ok2_OL SS1/updateSequencePhC/pol_ix1 ==
  note: 75dig -> 3iac
  ix : Inport
  Trigger : TriggerPort  TriggerType=function-call  VariantControl=(inherit)  PortDimensions=1
  If : If  IfExpression="(u1 > -8)  & (u1 < 8)"  ElseIfExpressions=u1 >= 8
  Merge : Merge  Inputs=3
  neg : Subsystem  TreatAsAtomicUnit=on
  pos : Subsystem  TreatAsAtomicUnit=on
  zero : Subsystem  TreatAsAtomicUnit=on
  pol_ix : Outport
  wires:
  Merge/1 -> pol_ix/1
  pos/1(Out1) -> Merge/2
  neg/1(Out1) -> Merge/3
  If/3 -> neg/Action
  If/2 -> pos/Action
  zero/1(Out1) -> Merge/1
  If/1 -> zero/Action
  ix/1 -> If/1

== system npc_controller/CONTROL/STATE-MACHINE/CPU_CONTROL_200_A2_precharge_pfc_ok2_OL SS1/updateSequencePhC/pol_vxn1 ==
  note: 16dig -> 5vac
  vxn : Inport
  ixn : Inport  Port=2
  Trigger : TriggerPort  TriggerType=function-call  VariantControl=(inherit)  PortDimensions=1
  If : If  IfExpression="(u1 > -16)  & (u1 < 16)"  ElseIfExpressions=u1 >= 16
  Merge : Merge  Inputs=3
  neg : Subsystem  TreatAsAtomicUnit=on
  pos : Subsystem  TreatAsAtomicUnit=on
  zero : Subsystem  TreatAsAtomicUnit=on
  pol_vxn : Outport
  wires:
  vxn/1 -> If/1
  If/1 -> zero/Action
  zero/1(Out1) -> Merge/1
  If/2 -> pos/Action
  If/3 -> neg/Action
  neg/1(Out1) -> Merge/3
  pos/1(Out1) -> Merge/2
  Merge/1 -> pol_vxn/1
  ixn/1 -> neg/1(ixn), pos/1(ixn)

== system npc_controller/CONTROL/STATE-MACHINE/CPU_CONTROL_200_A2_precharge_pfc_ok2_OL SS1/updateSequencePhC/pol_vxn2 ==
  note: 16dig -> 5vac
  vxn : Inport
  Trigger : TriggerPort  TriggerType=function-call  VariantControl=(inherit)  PortDimensions=1
  If : If  IfExpression="(u1 > -16)  & (u1 < 16)"  ElseIfExpressions=u1 >= 16
  Merge : Merge  Inputs=3
  neg : Subsystem  TreatAsAtomicUnit=on
  pos : Subsystem  TreatAsAtomicUnit=on
  zero : Subsystem  TreatAsAtomicUnit=on
  pol_vxn : Outport
  wires:
  Merge/1 -> pol_vxn/1
  pos/1(Out1) -> Merge/2
  neg/1(Out1) -> Merge/3
  If/3 -> neg/Action
  If/2 -> pos/Action
  zero/1(Out1) -> Merge/1
  If/1 -> zero/Action
  vxn/1 -> If/1

== system npc_controller/CONTROL/STATE-MACHINE/CPU_CONTROL_200_Vpk/configFutDis/System Outputs1 ==

== system npc_controller/CONTROL/STATE-MACHINE/CPU_CONTROL_200_Vpk/configFutDis/System Outputs2 ==

== system npc_controller/CONTROL/STATE-MACHINE/CPU_CONTROL_200_Vpk/configFutEn/System Outputs1 ==

== system npc_controller/CONTROL/STATE-MACHINE/CPU_CONTROL_200_Vpk/configFutEn/System Outputs2 ==

== system npc_controller/CONTROL/STATE-MACHINE/CPU_CONTROL_200_Vpk/configFutEn/System Outputs3 ==

== system npc_controller/CONTROL/STATE-MACHINE/CPU_CONTROL_200_Vpk/configGrid/FORCE_TZ ==
  note: 0 - Three phase
      | 1 - Single phase
  In1 : Inport
  sinlgeph_config : Inport  Port=2
  Trigger : TriggerPort  TriggerType=function-call  VariantControl=(inherit)  PortDimensions=1
  1P : Subsystem  TreatAsAtomicUnit=on
  3P3W : Subsystem  TreatAsAtomicUnit=on
  If : If  IfExpression=u1 == 0
  wires:
  If/1 -> 3P3W/Action
  sinlgeph_config/1 -> 1P/1(sinlgeph_config)
  If/2 -> 1P/Action
  In1/1 -> If/1

== system npc_controller/CONTROL/STATE-MACHINE/CPU_CONTROL_200_Vpk/configGrid/RESET_TZ ==
  note: EALLOW;
      |
      | /*Disabled tripzone action*/
      | EPwm6Regs.TZCTL.bit.TZA = (uint16_T)(0b11); //do nothing
      | EPwm6Regs.TZCTL.bit.TZB = (uint16_T)(0b11);
      | EPwm7Regs.TZCTL.bit.TZA = (uint16_T)(0b11);
      | EPwm7Regs.TZCTL.bit.TZB = (uint16_T)(0b11);
      | EPwm8Regs.TZCTL.bit.TZA = (uint16_T)(0b11);
      | EPwm8Regs.TZCTL.bit.TZB = (uint16_T)(0b11);
      | EPwm9Regs.TZCTL.bit.TZA = (uint16_T)(0b11);
      | EPwm9Regs.TZCTL.bit.TZB = (uint16_T)(0b11);
      | EPwm10Regs.TZCTL.bit.TZA = (uint16_T)(0b11);
      | EPwm10Regs.TZCTL.bit.TZB = (uint16_T)(0b11);
      | EPwm11Regs.TZCTL.bit.TZA = (uint16_T)(0b11);
      | EPwm11Regs.TZCTL.bit.TZB = (uint16_T)(0b11);
      |
      | /*Clear grouped OST TZ flags*/
      | EPwm6Regs.TZCLR.bit.OST = 0b1; //clear trip
      | EPwm7Regs.TZCLR.bit.OST = 0b1;
      | EPwm8Regs.TZCLR.bit.OST = 0b1;
      | EPwm9Regs.TZCLR.bit.OST = 0b1;
      | EPwm10Regs.TZCLR.bit.OST = 0b1;
      | EPwm11Regs.TZCLR.bit.OST = 0b1;
      |
      | /*Clear individual OST TZ flags*/
      | EPwm6Regs.TZOSTCLR.bit.OST1 = 0b1; //clear trip
      | EPwm6Regs.TZOSTCLR.bit.OST2 = 0b1;
      | EPwm7Regs.TZOSTCLR.bit.OST1 = 0b1;
      | EPwm7Regs.TZOSTCLR.bit.OST2 = 0b1;
      | EPwm8Regs.TZOSTCLR.bit.OST1 = 0b1;
      | EPwm8Regs.TZOSTCLR.bit.OST2 = 0b1;
      | EPwm9Regs.TZOSTCLR.bit.OST1 = 0b1;
      | EPwm9Regs.TZOSTCLR.bit.OST2 = 0b1;
      | EPwm10Regs.TZOSTCLR.bit.OST1 = 0b1;
      | EPwm10Regs.TZOSTCLR.bit.OST2 = 0b1;
      | EPwm11Regs.TZOSTCLR.bit.OST1 = 0b1;
      | EPwm11Regs.TZOSTCLR.bit.OST2 = 0b1;
      |
      | /*Enable tripzone action*/
      | EPwm6Regs.TZCTL.bit.TZA = (uint16_T)(0b10); //force to LOW
      | EPwm6Regs.TZCTL.bit.TZB = (uint16_T)(0b10);
      | EPwm7Regs.TZCTL.bit.TZA = (uint16_T)(0b10);
      | EPwm7Regs.TZCTL.bit.TZB = (uint16_T)(0b10);
      | EPwm8Regs.TZCTL.bit.TZA = (uint16_T)(0b10);
      | EPwm8Regs.TZCTL.bit.TZB = (uint16_T)(0b10);
      | EPwm9Regs.TZCTL.bit.TZA = (uint16_T)(0b10);
      | EPwm9Regs.TZCTL.bit.TZB = (uint16_T)(0b10);
      | EPwm10Regs.TZCTL.bit.TZA = (uint16_T)(0b10);
      | EPwm10Regs.TZCTL.bit.TZB = (uint16_T)(0b10);
      | EPwm11Regs.TZCTL.bit.TZA = (uint16_T)(0b10);
      | EPwm11Regs.TZCTL.bit.TZB = (uint16_T)(0b10);
      |
      | EDIS;
  note: Note:
      | TZCCTL
      | 0b00 - High impedance
      | 0b01 - Force to HIGH
      | 0b10 - Force to LOW
      | 0b11 - Do nothing
      |
      | AQCSFRC
      | 0b00 - disables forced PWM
      | 0b01 - forces PWM to LOW
      | 0b10 - forces PWM to  HIGH
      |
      | TZFRC.bit.OST
      | 0b0 - Do nothing
      | 0b1 - Force TZ
  Trigger : TriggerPort  TriggerType=function-call  VariantControl=(inherit)  PortDimensions=1
  System Outputs2 : Subsystem  mask(System Outputs){ShowInLibBrowser=0}
      mask prompts: ShowInLibBrowser "Simulink:masks:CustCodeMaskParam1_MP"
      settings: CopyFcn=cccopyfcn(gcb)  OpenFcn=ccopenfcn('System Outputs Function')
      mask Help: eval('feval(''rtwprivate'',''rtwhelpview'',''rtw_sys_outputs_block'')');
      mask Display: disp('System\nOutputs');

== system npc_controller/CONTROL/STATE-MACHINE/CPU_CONTROL_200_Vpk/detectUvpOvp/false ==
  Action Port : ActionPort
  Constant1 : Constant  OutDataTypeStr=boolean  SampleTime=-1
  high : Outport
  wires:
  Constant1/1 -> high/1

== system npc_controller/CONTROL/STATE-MACHINE/CPU_CONTROL_200_Vpk/detectUvpOvp/true ==
  Action Port : ActionPort
  Constant : Constant  Value=0  OutDataTypeStr=boolean  SampleTime=-1
  low : Outport
  wires:
  Constant/1 -> low/1

== system npc_controller/CONTROL/STATE-MACHINE/CPU_CONTROL_200_Vpk/detectZCPhA/false ==
  Action Port : ActionPort
  Constant1 : Constant  Value=0  OutDataTypeStr=boolean  SampleTime=-1
  ph_en_out : Outport
  wires:
  Constant1/1 -> ph_en_out/1

== system npc_controller/CONTROL/STATE-MACHINE/CPU_CONTROL_200_Vpk/detectZCPhA/true ==
  Action Port : ActionPort
  Constant : Constant  OutDataTypeStr=boolean  SampleTime=-1
  ph_en : Outport
  wires:
  Constant/1 -> ph_en/1

== system npc_controller/CONTROL/STATE-MACHINE/CPU_CONTROL_200_Vpk/detectZCPhB/false ==
  Action Port : ActionPort
  Constant1 : Constant  Value=0  OutDataTypeStr=boolean  SampleTime=-1
  ph_en_out : Outport
  wires:
  Constant1/1 -> ph_en_out/1

== system npc_controller/CONTROL/STATE-MACHINE/CPU_CONTROL_200_Vpk/detectZCPhB/true ==
  Action Port : ActionPort
  Constant : Constant  OutDataTypeStr=boolean  SampleTime=-1
  ph_en : Outport
  wires:
  Constant/1 -> ph_en/1

== system npc_controller/CONTROL/STATE-MACHINE/CPU_CONTROL_200_Vpk/detectZCPhC/false ==
  Action Port : ActionPort
  Constant1 : Constant  Value=0  OutDataTypeStr=boolean  SampleTime=-1
  ph_en_out : Outport
  wires:
  Constant1/1 -> ph_en_out/1

== system npc_controller/CONTROL/STATE-MACHINE/CPU_CONTROL_200_Vpk/detectZCPhC/true ==
  Action Port : ActionPort
  Constant : Constant  OutDataTypeStr=boolean  SampleTime=-1
  ph_en : Outport
  wires:
  Constant/1 -> ph_en/1

== system npc_controller/CONTROL/STATE-MACHINE/CPU_CONTROL_200_Vpk/disDigCmpMode/System Outputs2 ==

== system npc_controller/CONTROL/STATE-MACHINE/CPU_CONTROL_200_Vpk/disablePwm/System Outputs ==

== system npc_controller/CONTROL/STATE-MACHINE/CPU_CONTROL_200_Vpk/enDigCmpMode/System Outputs2 ==

== system npc_controller/CONTROL/STATE-MACHINE/CPU_CONTROL_200_Vpk/updateCalib/cnt ==
  cnt_calib : Inport  OutDataTypeStr=uint16
  van : Inport  Port=2  OutDataTypeStr=single  PortDimensions=1
  vbn : Inport  Port=3  OutDataTypeStr=single  PortDimensions=1
  vcn : Inport  Port=4  OutDataTypeStr=single  PortDimensions=1
  ia : Inport  Port=5  OutDataTypeStr=single  PortDimensions=1
  ib : Inport  Port=6  OutDataTypeStr=single  PortDimensions=1
  ic : Inport  Port=7  OutDataTypeStr=single  PortDimensions=1
  Action Port : ActionPort
  Add : Sum  AccumDataTypeStr=uint16  OutDataTypeStr=uint16
  Constant : Constant  OutDataTypeStr=uint16  SampleTime=-1
  Constant1 : Constant  Value=0  OutDataTypeStr=boolean  SampleTime=-1
  Data Store Write : DataStoreWrite  DataStoreName=adc_offset_ib_tmp  IndexOptions=Index vector (dialog)  Indices=1  OutputSizes=1
  Data Store Write1 : DataStoreWrite  DataStoreName=adc_offset_ic_tmp  IndexOptions=Index vector (dialog)  Indices=1  OutputSizes=1
  Data Store Write2 : DataStoreWrite  DataStoreName=cnt_calib  IndexOptions=Index vector (dialog)  Indices=1  OutputSizes=1
  Data Store Write3 : DataStoreWrite  DataStoreName=adc_offset_vc_tmp  IndexOptions=Index vector (dialog)  Indices=1  OutputSizes=1
  Data Store Write4 : DataStoreWrite  DataStoreName=adc_offset_ia_tmp  IndexOptions=Index vector (dialog)  Indices=1  OutputSizes=1
  Data Store Write5 : DataStoreWrite  DataStoreName=adc_offset_va_tmp  IndexOptions=Index vector (dialog)  Indices=1  OutputSizes=1
  Data Store Write6 : DataStoreWrite  DataStoreName=adc_offset_vb_tmp  IndexOptions=Index vector (dialog)  Indices=1  OutputSizes=1
  IIR Filter2 : Subsystem  Commented=on
  Subsystem1 : Subsystem
  Subsystem2 : Subsystem
  Subsystem3 : Subsystem
  Subsystem4 : Subsystem
  Subsystem5 : Subsystem
  Subsystem6 : Subsystem
  calib_ok : Outport
  wires:
  cnt_calib/1 -> Add/1
  Add/1 -> Data Store Write2/1
  Constant1/1 -> calib_ok/1
  Subsystem2/1(average) -> Data Store Write/1  "va"
  Constant/1 -> Add/2
  Subsystem1/1(average) -> Data Store Write1/1  "va"
  Subsystem3/1(average) -> Data Store Write4/1  "va"
  Subsystem4/1(average) -> Data Store Write3/1  "va"
  Subsystem6/1(average) -> Data Store Write5/1  "va"
  van/1 -> Subsystem6/1(sample)
  Subsystem5/1(average) -> Data Store Write6/1  "va"
  vcn/1 -> Subsystem4/1(sample)
  vbn/1 -> Subsystem5/1(sample)
  ia/1 -> Subsystem3/1(sample)
  ic/1 -> Subsystem1/1(sample)
  ib/1 -> Subsystem2/1(sample)

== system npc_controller/CONTROL/STATE-MACHINE/CPU_CONTROL_200_Vpk/updateCalib/done ==
  Action Port : ActionPort
  AUTO-CALIB_DONE : Subsystem
  CLEAR_FAULTS : Subsystem
  Function-Call Generator : simulink/Ports & Subsystems/Function-Call Generator  sample_time=-1  numberOfIterations=1  DisallowWideOutput=off
  Function-Call Split1 : FunctionCallSplit  NumOutputPorts=2
  Function-Call Split2 : FunctionCallSplit  NumOutputPorts=2
  RESET_TZ : Subsystem
  calib_ok : Outport
  wires:
  Function-Call Generator/1 -> Function-Call Split1/1
  Function-Call Split1/2 -> Function-Call Split2/1
  AUTO-CALIB_DONE/1(Out1) -> calib_ok/1
  Function-Call Split1/1 -> AUTO-CALIB_DONE/Trigger
  Function-Call Split2/1 -> RESET_TZ/Trigger
  Function-Call Split2/2 -> CLEAR_FAULTS/Trigger
